simulink model "twoSpecies_LV_Sim"  (R2019b)
settings: Solver=FixedStepAuto  StartTime=0.0  StopTime=10  FixedStep=0.01  RelTol=1e-3
settings Model: Creator=cristian  LastModifiedBy=cristian

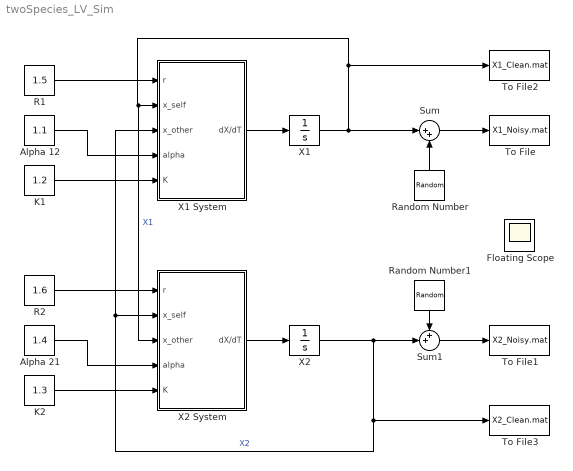
== system twoSpecies_LV_Sim ==
  Alpha 12 : Constant  Value=1.1
  Alpha 21 : Constant  Value=1.4
  Floating Scope : Scope
      settings: Floating=on
  K1 : Constant  Value=1.2
  K2 : Constant  Value=1.3
  R1 : Constant  Value=1.5
  R2 : Constant  Value=1.6
  Random Number : RandomNumber  Variance=0.0001  SampleTime=0.01
  Random Number1 : RandomNumber  Variance=0.0001  SampleTime=0.01
  Sum : Sum  Inputs=|++
  Sum1 : Sum  Inputs=++|
  To File : ToFile  Filename=X1_Noisy.mat  MatrixName=speciesOne_Noisy
  To File1 : ToFile  Filename=X2_Noisy.mat  MatrixName=speciesTwo_Noisy
  To File2 : ToFile  Filename=X1_Clean.mat  MatrixName=speciesOne_Clean
  To File3 : ToFile  Filename=X2_Clean.mat  MatrixName=speciesTwo_Clean
  X1 : Integrator  InitialCondition=0.01  LimitOutput=on  LowerSaturationLimit=0
  X1 System : Subsystem
  X2 : Integrator  InitialCondition=0.02  LimitOutput=on  LowerSaturationLimit=0
  X2 System : Subsystem
  wires:
  X1 System/1(dX/dT) -> X1/1
  X2 System/1(dX/dT) -> X2/1
  X1/1 -> To File2/1, X2 System/3(x_other), X1 System/2(x_self), Sum/1  "X1"
  R1/1 -> X1 System/1(r)
  Alpha 12/1 -> X1 System/4(alpha)
  K1/1 -> X1 System/5(K)
  K2/1 -> X2 System/5(K)
  Alpha 21/1 -> X2 System/4(alpha)
  R2/1 -> X2 System/1(r)
  Sum/1 -> To File/1
  Random Number/1 -> Sum/2
  Random Number1/1 -> Sum1/1
  Sum1/1 -> To File1/1
  X2/1 -> To File3/1, X1 System/3(x_other), X2 System/2(x_self), Sum1/2  "X2"

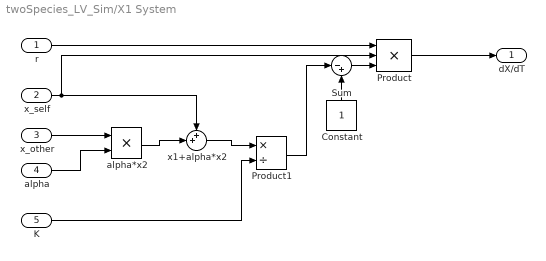
== system twoSpecies_LV_Sim/X1 System ==
  r : Inport
  x_self : Inport  Port=2
  x_other : Inport  Port=3
  alpha : Inport  Port=4
  K : Inport  Port=5
  Constant : Constant
  Product : Product  Inputs=3
  Product1 : Product  Inputs=*/
  Sum : Sum  Inputs=|-+
  alpha*x2 : Product
  x1+alpha*x2 : Sum  Inputs=++|
  dX/dT : Outport
  wires:
  x1+alpha*x2/1 -> Product1/1
  Constant/1 -> Sum/2
  Sum/1 -> Product/3
  K/1 -> Product1/2
  Product/1 -> dX/dT/1
  Product1/1 -> Sum/1
  x_other/1 -> alpha*x2/1
  x_self/1 -> x1+alpha*x2/1, Product/2
  alpha*x2/1 -> x1+alpha*x2/2
  alpha/1 -> alpha*x2/2
  r/1 -> Product/1

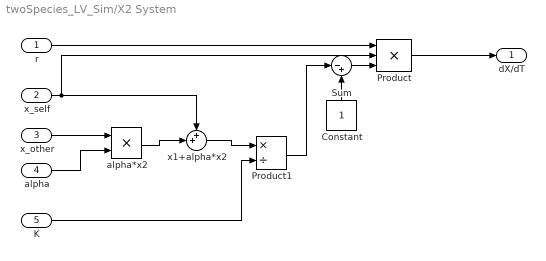
== system twoSpecies_LV_Sim/X2 System ==
  r : Inport
  x_self : Inport  Port=2
  x_other : Inport  Port=3
  alpha : Inport  Port=4
  K : Inport  Port=5
  Constant : Constant
  Product : Product  Inputs=3
  Product1 : Product  Inputs=*/
  Sum : Sum  Inputs=|-+
  alpha*x2 : Product
  x1+alpha*x2 : Sum  Inputs=++|
  dX/dT : Outport
  wires:
  x1+alpha*x2/1 -> Product1/1
  Constant/1 -> Sum/2
  Sum/1 -> Product/3
  K/1 -> Product1/2
  Product/1 -> dX/dT/1
  Product1/1 -> Sum/1
  x_other/1 -> alpha*x2/1
  x_self/1 -> x1+alpha*x2/1, Product/2
  alpha*x2/1 -> x1+alpha*x2/2
  alpha/1 -> alpha*x2/2
  r/1 -> Product/1
